simulink model "actuatorModel"  (R2018b)
settings: Solver=VariableStepAuto  StartTime=0.0  StopTime=10.0  RelTol=1e-3
model workspace (MAT data in the model file):
  actuatorCentres.aileron.left = 0
  actuatorCentres.aileron.right = 0
  actuatorCentres.elevator.left = 0
  actuatorCentres.elevator.right = 0
  actuatorCentres.rudder = 0
  actuatorCentres.flap.left = 0
  actuatorCentres.flap.right = 0
  deflectionLimits.aileron.min = -10
  deflectionLimits.aileron.max = 10
  deflectionLimits.elevator.min = -10
  deflectionLimits.elevator.max = 10
  deflectionLimits.rudder.min = -5
  deflectionLimits.rudder.max = 5
  deflectionLimits.flap.min = 0
  deflectionLimits.flap.max = 15
  servoPins.aileron.left = 9
  servoPins.aileron.right = 10
  servoPins.elevator.left = 7
  servoPins.elevator.right = 8
  servoPins.rudder = 11
  servoPins.flap.left = 5
  servoPins.flap.right = 6
values from neighbouring files (symbols this model uses):
  actuatorCentres = 0.0    [data.sldd]
  deflectionLimits = -10.0    [data.sldd]
libraries: arduinolib x7
settings Model: OrderedModelArguments=off  Creator=Aliak  LastModifiedBy=Aliak

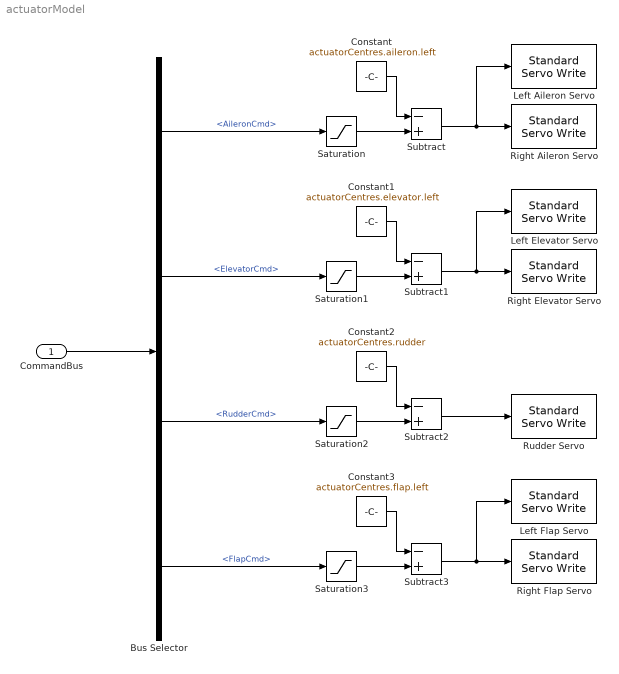
== system actuatorModel ==
  CommandBus : Inport
  Bus Selector : BusSelector  OutputSignals=AileronCmd,ElevatorCmd,RudderCmd,FlapCmd
  Constant : Constant  Value=actuatorCentres.aileron.left
  Constant1 : Constant  Value=actuatorCentres.elevator.left
  Constant2 : Constant  Value=actuatorCentres.rudder
  Constant3 : Constant  Value=actuatorCentres.flap.left
  Left Aileron Servo : arduinolib/Standard Servo Write  pinNumber=servoPins.aileron.left  ServoIndex=0  blockPlatform=ARDUINO
      settings: SourceProductName=Simulink Support Package for Arduino Hardware
  Left Elevator Servo : arduinolib/Standard Servo Write  pinNumber=servoPins.elevator.left  ServoIndex=0  blockPlatform=ARDUINO
      settings: SourceProductName=Simulink Support Package for Arduino Hardware
  Left Flap Servo : arduinolib/Standard Servo Write  pinNumber=servoPins.flap.left  ServoIndex=0  blockPlatform=ARDUINO
      settings: SourceProductName=Simulink Support Package for Arduino Hardware
  Right Aileron Servo : arduinolib/Standard Servo Write  pinNumber=servoPins.aileron.right  ServoIndex=0  blockPlatform=ARDUINO
      settings: SourceProductName=Simulink Support Package for Arduino Hardware
  Right Elevator Servo : arduinolib/Standard Servo Write  pinNumber=servoPins.elevator.right  ServoIndex=0  blockPlatform=ARDUINO
      settings: SourceProductName=Simulink Support Package for Arduino Hardware
  Right Flap Servo : arduinolib/Standard Servo Write  pinNumber=servoPins.flap.right  ServoIndex=0  blockPlatform=ARDUINO
      settings: SourceProductName=Simulink Support Package for Arduino Hardware
  Rudder Servo : arduinolib/Standard Servo Write  pinNumber=servoPins.rudder  ServoIndex=0  blockPlatform=ARDUINO
      settings: SourceProductName=Simulink Support Package for Arduino Hardware
  Saturation : Saturate  UpperLimit=deflectionLimits.aileron.max  LowerLimit=deflectionLimits.aileron.min
  Saturation1 : Saturate  UpperLimit=deflectionLimits.elevator.max  LowerLimit=deflectionLimits.elevator.min
  Saturation2 : Saturate  UpperLimit=deflectionLimits.rudder.max  LowerLimit=deflectionLimits.rudder.min
  Saturation3 : Saturate  UpperLimit=deflectionLimits.flap.max  LowerLimit=deflectionLimits.flap.min
  Subtract{,1..3} (4 alike) : Sum  Inputs=-+
  wires:
  CommandBus/1 -> Bus Selector/1
  Bus Selector/1 -> Saturation/1  "<AileronCmd>"
  Bus Selector/2 -> Saturation1/1  "<ElevatorCmd>"
  Bus Selector/3 -> Saturation2/1  "<RudderCmd>"
  Bus Selector/4 -> Saturation3/1  "<FlapCmd>"
  Constant/1 -> Subtract/1
  Saturation/1 -> Subtract/2
  Subtract/1 -> Right Aileron Servo/1, Left Aileron Servo/1
  Subtract1/1 -> Right Elevator Servo/1, Left Elevator Servo/1
  Saturation1/1 -> Subtract1/2
  Constant1/1 -> Subtract1/1
  Subtract2/1 -> Rudder Servo/1
  Saturation2/1 -> Subtract2/2
  Constant2/1 -> Subtract2/1
  Subtract3/1 -> Right Flap Servo/1, Left Flap Servo/1
  Saturation3/1 -> Subtract3/2
  Constant3/1 -> Subtract3/1
